simulink model "suspension"  (R2024a)
settings: Solver=FixedStepAuto  StartTime=0.0  StopTime=20  RelTol=1e-3  EnableMultiTasking=on
undefined symbols (not defined in the file): Green, led0
libraries: raspberrypiBasiclib x4
settings Model: Creator=mikom  LastModifiedBy=mikom
settings SolverCC: PositivePriorityOrder=on
settings OptimizationCC: EnhancedBackFolding=on  PassReuseOutputArgsAs=Individual arguments  ZeroExternalMemoryAtStartup=off  ZeroInternalMemoryAtStartup=off  MaxStackSize=64  OptimizeBlockOrder=speed  DifferentSizesBufferReuse=on  OptimizationCustomize=off  EfficientTunableParamExpr=on
settings DebuggingCC: ParameterTunabilityLossMsg=error
settings HardwareCC: ProdBitPerPointer=32  ProdBitPerSizeT=32  ProdBitPerPtrDiffT=32  ProdLargestAtomicInteger=Long  ProdLargestAtomicFloat=Double  ProdWordSize=32  ProdLongLongMode=on  ProdHWDeviceType=ARM Compatible->ARM Cortex
settings RTWCC: Description=Embedded Coder  SystemTargetFile=ert.tlc  HardwareBoard=Raspberry Pi  TLCOptions="-aInlineSetEventsForThisBaseRateFcn=TLC_FALSE -aSuppressMultiTaskScheduler=TLC_FALSE  -aRateBasedStepFcn=0"  TemplateMakefile=ert_default_tmf  Toolchain=GNU GCC Embedded Linux  BuildConfiguration=Faster Runs
settings CodeAppCC: ForceParamTrailComments=on  IgnoreCustomStorageClasses=off  OperatorAnnotations=on  SimulinkDataObjDesc=on  SFDataObjDesc=on  InsertBlockDesc=on
settings ERTTargetCC: MatFileLogging=on  SupportContinuousTime=on  SupportVariableSizeSignals=on  ExtModeTransport=2  ExtModeStaticAlloc=on  ExtModeMexFile=ext_xcp  ExtModeIntrfLevel=Level2 - Open

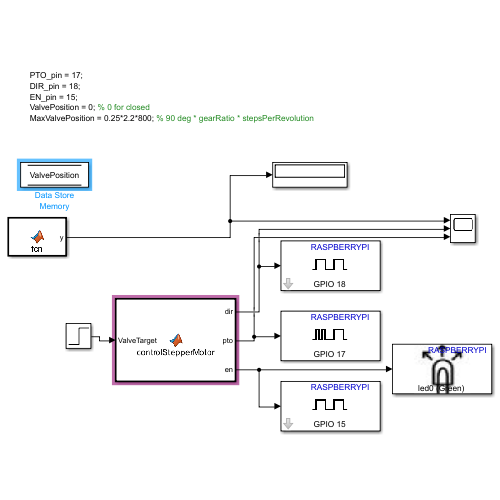
[thumbnail: Simulink's stored preview of the top-level diagram]
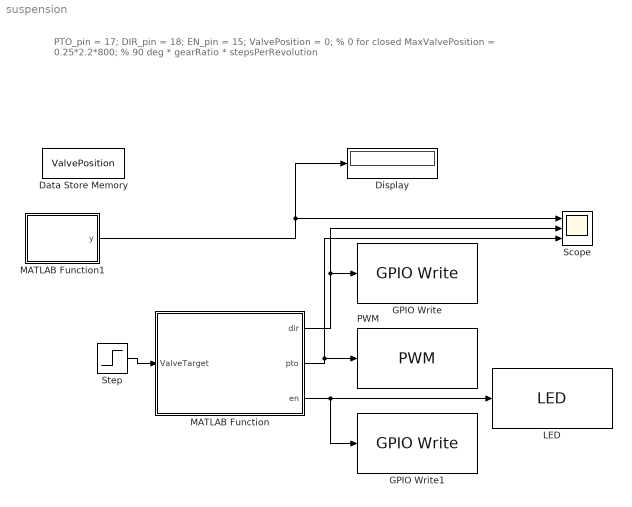
== system suspension ==
  note: PTO_pin = 17;
      | DIR_pin = 18;
      | EN_pin = 15;
      | ValvePosition = 0; % 0 for closed
      | MaxValvePosition = 0.25*2.2*800; % 90 deg * gearRatio * stepsPerRevolution
  Data Store Memory : DataStoreMemory  DataStoreName=ValvePosition  WriteAfterWriteMsg=warning  InitialValue=ValvePosition  ShowAdditionalParam=off  OutDataTypeStr=int16
  Display : Display
  GPIO Write : raspberrypiBasiclib/GPIO Write  board=Pi 4 Model B  gpio=18  direction=Output  blockPlatform=Raspberry Pi
  GPIO Write1 : raspberrypiBasiclib/GPIO Write  board=Pi 4 Model B  gpio=15  direction=Output  blockPlatform=Raspberry Pi
  LED : raspberrypiBasiclib/LED  BoardProperty=Pi 4 Model B  LED_=led0 (Green)
  MATLAB Function : MATLAB Function  TreatAsAtomicUnit=on
  MATLAB Function1 : MATLAB Function  TreatAsAtomicUnit=on
  PWM : raspberrypiBasiclib/PWM  board=Pi 4 Model B  Pin_=17  Frequency=100  blockPlatform=Raspberry Pi
  Scope : Scope  NumInputPorts=3
  Step : Step  Time=2  After=100  SampleTime=0
  wires:
  Step/1 -> MATLAB Function/1(ValveTarget)
  MATLAB Function/1(dir) -> Scope/2, GPIO Write/1
  MATLAB Function/3(en) -> LED/1, GPIO Write1/1
  MATLAB Function/2(pto) -> Scope/3, PWM/1
  MATLAB Function1/1(y) -> Display/1, Scope/1

== matlab function suspension/MATLAB Function1 ==
  data: y output
function y = fcn()
global ValvePosition,
y = ValvePosition;

== matlab function suspension/MATLAB Function ==
  data: ValveTarget input; dir output; pto output; en output; ValvePosition data_store_memory
function [dir, pto, en] = controlStepperMotor(ValveTarget)
    Speed = 0.5;
    % Determine the direction based on the valve position
    global ValvePosition,
    if ValvePosition > ValveTarget
        dir = 1; % closing
        en = 1;
        pto = Speed;
        ValvePosition=ValvePosition-1;
    else if ValvePosition < ValveTarget
        dir = 0; % opening
        en = 1;
        pto = Speed;
        ValvePosition=ValvePosition+1;
    else
        dir = 0; % in position
        en = 0;
        pto = 0;
    end
end
